simulink library "Energy_converter_Electrical_to_Mechanical"  (R2016a)
settings: Solver=ode1  StartTime=0.0  StopTime=Inf  FixedStep=0.001  RelTol=1e-3
undefined symbols (not defined in the file): API1dcac_efficiency, API2dcac_efficiency, API3dcac_efficiency, aux_power_state, AWR_InvStError, dat, DiscIntNeverNeededParam, EDCU_p_RefTqeMOT, emot_AcCmprFront_inertia, emot_AcCmprFront_nTab_3rdD, emot_AcCmprFront_pwrAC, emot_AcCmprFront_Tau, emot_AcCmprFront_trqTab_2ndD, emot_AcCmprFront_vltTab_1stD, emot_AcCmprRear_inertia, emot_AcCmprRear_nTab_3rdD, emot_AcCmprRear_pwrAC, emot_AcCmprRear_Tau, emot_AcCmprRear_trqTab_2ndD, emot_AcCmprRear_vltTab_1stD, emot_AirCmpr_inertia, emot_AirCmpr_nTab_3rdD, emot_AirCmpr_pwrAC, emot_AirCmpr_Tau, emot_AirCmpr_trqTab_2ndD, emot_AirCmpr_vltTab_1stD, emot_aircomp_power, emot_Cth_rotor, emot_Cth_stator, emot_dtrqEmotNeg, emot_dtrqEmotPtv, emot_inv_pwracTab_1st, emot_inv_pwrDC, emot_inv_pwrLoss, emot_inv_VrmsTab_2nd, emot_j, emot_mot_pwrLoss, emot_nTab_1stD, emot_pwrEtaTab_nRow, emot_pwrEtaTab_pwrTab, emot_pwrEtaTab_trqClm, emot_Rth_rotor_oil, emot_Rth_stator_oil, emot_Rth_stator_rotor, emot_tractiongroup, emot_Trotor_init, emot_trqMaxRow, emot_trqMinRow, emot_Tstator_init, emot_vltTab_3rdD, FirstDrivenAxleNoOfEmot, inv_Cth_cooling_plate, inv_Cth_diode, inv_Cth_IGBT, inv_n_IGBT_per_Switch, inv_Rth_cooling_plate_coolant, inv_Rth_PS_cooling_plate, inv_Tplate_init, inv_Tpowerstack_init, midAxleNoOfEmot ... (+6)
libraries: Electrical_converter x12, Energy_converter_Electrical_to_Mechanical x12, simulink x7
(part 8 of 8)

== system Energy_converter_Electrical_to_Mechanical/e-Motor_chy_proposal/Umrichter mit trq-Regler/Rate Limiter Dynamic/Saturation Dynamic ==
  up : Inport
  u : Inport  Port=2
  lo : Inport  Port=3
  Data Type Duplicate : DataTypeDuplicate  DisableCoverage=on
  Data Type Propagation : S-Function  FunctionName=sfix_dtprop  Parameters=14,PropDataTypeMode,(getdatatypespecs(PropDataType,PropScaling,DblOver,0, 0, PropDataTypeMode, PropScalingMode)),IfRefDouble,IfRefSingle,IsSigned,NumBitsBase,NumBitsMult,NumBitsAdd,(sort(reshape(round(NumBitsAllowFinal), prod(size(NumBitsAllowFinal)),1))),PropScalingMode,ValuesUsedBestPrec,SlopeBase,SlopeMult,SlopeAdd,BiasBase,BiasMult,BiasAdd,DblOver  SFunctionDeploymentMode=off  EnableBusSupport=off  mask(Data Type Propagation){PropDataTypeMode=Inherit via propagation rule, PropDataType=fixdt(1, 16), IfRefDouble=double, IfRefSingle=single, IsSigned=IsSigned1, NumBitsBase=NumBits1, NumBitsMult=1, NumBitsAdd=0, NumBitsAllowFinal=1:128, PropScalingMode=Inherit via propagation rule, PropScaling=2^-10, ValuesUsedBestPrec=[5 -7], SlopeBase=Slope1, SlopeMult=1, SlopeAdd=0, BiasBase=Bias1, BiasMult=1, BiasAdd=0}
      mask prompts: PropDataTypeMode "Simulink:masks:x1PropagatedDataType_MP"; PropDataType "Simulink:masks:x11PropagatedDataTypeegFixdt116Fixdtsingle_MP"; IfRefDouble "Simulink:masks:x11IfAnyReferenceInputIsDoubleOutputIs_MP"; IfRefSingle "Simulink:masks:x12IfAnyReferenceInputIsSingleOutputIs_MP"; IsSigned "Simulink:masks:x13IsSigned_MP"; NumBitsBase "Simulink:masks:x141NumberofBitsBase_MP"; NumBitsMult "Simulink:masks:x142NumberofBitsMultiplicativeAdjustment_MP"; NumBitsAdd "Simulink:masks:x143NumberofBitsAdditiveAdjustment_MP"; NumBitsAllowFinal "Simulink:masks:x144NumberofBitsAllowableFinalValues_MP"; PropScalingMode "Simulink:masks:x2PropagatedScaling_MP"; PropScaling "Simulink:masks:x21PropagatedScalingSlopeEg29OrSlopeBiasEg1253_MP"; ValuesUsedBestPrec "Simulink:masks:x21ValuesUsedToDetermineBestPrecisionScaling_MP"; SlopeBase "Simulink:masks:x211SlopeBase_MP"; SlopeMult "Simulink:masks:x212SlopeMultiplicativeAdjustment_MP"; SlopeAdd "Simulink:masks:x213SlopeAdditiveAdjustment_MP"; BiasBase "Simulink:masks:x221BiasBase_MP"; BiasMult "Simulink:masks:x222BiasMultiplicativeAdjustment_MP"; BiasAdd "Simulink:masks:x223BiasAdditiveAdjustment_MP"
      mask help: Simulink:masks:DataTypePropagation_MD
      mask init:
      | DblOver = 0;
      mask TypeOptions PropDataTypeMode: Simulink:masks:SpecifyViaDialog | Simulink:masks:InheritViaPropagationRule
      mask Callback PropDataTypeMode: fixptdialog(gcbh)
      mask Callback PropDataType: fixptdialog(gcbh)
      mask TypeOptions IfRefDouble: Simulink:masks:double | Simulink:masks:single
      mask TypeOptions IfRefSingle: Simulink:masks:double | Simulink:masks:single
      mask TypeOptions IsSigned: Simulink:masks:IsSigned1 | Simulink:masks:IsSigned2 | Simulink:masks:IsSigned1OrIsSigned2 | Simulink:masks:TRUE | Simulink:masks:FALSE
      mask TypeOptions NumBitsBase: NumBits1 | NumBits2 | max([NumBits1 NumBits2]) | min([NumBits1 NumBits2]) | NumBits1+NumBits2
      mask TypeOptions PropScalingMode: Simulink:masks:SpecifyViaDialog | Simulink:masks:InheritViaPropagationRule | Simulink:masks:ObtainViaBestPrecision
      mask Callback PropScalingMode: fixptdialog(gcbh)
      mask TypeOptions SlopeBase: Slope1 | Slope2 | max([Slope1 Slope2]) | min([Slope1 Slope2]) | Slope1*Slope2 | Slope1/Slope2 | PosRange1 | PosRange2 | max([PosRange1 PosRange2]) | min([PosRange1 PosRange2]) | PosRange1*PosRange2 | PosRange1/PosRange2
      mask TypeOptions BiasBase: Bias1 | Bias2 | max([Bias1 Bias2]) | min([Bias1 Bias2]) | Bias1*Bias2 | Bias1/Bias2 | Bias1+Bias2 | Bias1-Bias2
      mask Display:
      | port_label('Input',1,'Ref1');
      | port_label('Input',2,'Ref2');
      | port_label('Input',3,'Prop');
  LowerRelop1 : RelationalOperator  DisableCoverage=on  Operator=>  OutDataTypeStr=boolean
  Switch : Switch  Criteria=u2 ~= 0  OutDataTypeStr=Inherit: Inherit via back propagation  ZeroCross=off
  Switch2 : Switch  Criteria=u2 ~= 0  OutMin=OutMin  OutMax=OutMax  OutDataTypeStr=Inherit: Inherit via back propagation  ZeroCross=off
  UpperRelop : RelationalOperator  DisableCoverage=on  Operator=<  OutDataTypeStr=boolean
  y : Outport  OutMin=OutMin  OutMax=OutMax
  wires:
  up/1 -> Switch2/1, LowerRelop1/2
  u/1 -> Data Type Propagation/2, Data Type Propagation/1, LowerRelop1/1, Switch/3, UpperRelop/1
  lo/1 -> Switch/1, UpperRelop/2
  Switch/1 -> Data Type Duplicate/2, Switch2/3, Data Type Propagation/3
  Switch2/1 -> Data Type Duplicate/1, y/1
  LowerRelop1/1 -> Switch2/2
  UpperRelop/1 -> Switch/2

== matlab function Energy_converter_Electrical_to_Mechanical/AWR_DriveEmot_Gen2/MotorSelection/Truth Table ==
  data: u1 input; y1 output; u2 input; y2 output; y3 output; y4 output
function [y1, y2, y3, y4] = fcn(u1, u2)

aVarTruthTableCondition_1 = false;
aVarTruthTableCondition_2 = false;
aVarTruthTableCondition_3 = false;
aVarTruthTableCondition_4 = false;
aVarTruthTableCondition_5 = false;
aVarTruthTableCondition_6 = false;
aVarTruthTableCondition_7 = false;
aVarTruthTableCondition_8 = false;
aVarTruthTableCondition_9 = false;


% MidAxle - 0  and Rear Axle - 0 [One Powered Axle]

aVarTruthTableCondition_1 = logical(u1 == 0 && u2 == 0);

% MidAxle - 0  and Rear Axle - 1 [One Powered Axle]

aVarTruthTableCondition_2 = logical(u1 == 0 && u2 == 1);

% MidAxle - 0  and Rear Axle - 2 [One Powered Axle]

aVarTruthTableCondition_3 = logical(u1 == 0 && u2 == 2);

% MidAxle - 1  and Rear Axle - 0 [Two Powered Axle]

aVarTruthTableCondition_4 = logical(u1 == 1 && u2 == 0);

% MidAxle - 1  and Rear Axle - 1 [Two Powered Axle]

aVarTruthTableCondition_5 = logical(u1 == 1 && u2 == 1);

% MidAxle - 1  and Rear Axle - 2 [Two Powered Axle]

aVarTruthTableCondition_6 = logical(u1 == 1 && u2 == 2);

% MidAxle - 2  and Rear Axle - 0 [Two Powered Axle]

aVarTruthTableCondition_7 = logical(u1 == 2 && u2 == 0);

% MidAxle - 2  and Rear Axle - 1 [Two Powered Axle]

aVarTruthTableCondition_8 = logical(u1 == 2 && u2 == 1);

% MidAxle - 2  and Rear Axle - 2 [Two Powered Axle]

aVarTruthTableCondition_9 = logical(u1 == 2 && u2 == 2);

if (aVarTruthTableCondition_1 && ~aVarTruthTableCondition_2 && ~aVarTruthTableCondition_3 && ~aVarTruthTableCondition_4 && ~aVarTruthTableCondition_5 && ~aVarTruthTableCondition_6 && ~aVarTruthTableCondition_7 && ~aVarTruthTableCondition_8 && ~aVarTruthTableCondition_9)
    aFcnTruthTableAction_1();
elseif (~aVarTruthTableCondition_1 && aVarTruthTableCondition_2 && ~aVarTruthTableCondition_3 && ~aVarTruthTableCondition_4 && ~aVarTruthTableCondition_5 && ~aVarTruthTableCondition_6 && ~aVarTruthTableCondition_7 && ~aVarTruthTableCondition_8 && ~aVarTruthTableCondition_9)
    aFcnTruthTableAction_2();
elseif (~aVarTruthTableCondition_1 && ~aVarTruthTableCondition_2 && aVarTruthTableCondition_3 && ~aVarTruthTableCondition_4 && ~aVarTruthTableCondition_5 && ~aVarTruthTableCondition_6 && ~aVarTruthTableCondition_7 && ~aVarTruthTableCondition_8 && ~aVarTruthTableCondition_9)
    aFcnTruthTableAction_3();
elseif (~aVarTruthTableCondition_1 && ~aVarTruthTableCondition_2 && ~aVarTruthTableCondition_3 && aVarTruthTableCondition_4 && ~aVarTruthTableCondition_5 && ~aVarTruthTableCondition_6 && ~aVarTruthTableCondition_7 && ~aVarTruthTableCondition_8 && ~aVarTruthTableCondition_9)
    aFcnTruthTableAction_4();
elseif (~aVarTruthTableCondition_1 && ~aVarTruthTableCondition_2 && ~aVarTruthTableCondition_3 && ~aVarTruthTableCondition_4 && aVarTruthTableCondition_5 && ~aVarTruthTableCondition_6 && ~aVarTruthTableCondition_7 && ~aVarTruthTableCondition_8 && ~aVarTruthTableCondition_9)
    aFcnTruthTableAction_5();
elseif (~aVarTruthTableCondition_1 && ~aVarTruthTableCondition_2 && ~aVarTruthTableCondition_3 && ~aVarTruthTableCondition_4 && ~aVarTruthTableCondition_5 && aVarTruthTableCondition_6 && ~aVarTruthTableCondition_7 && ~aVarTruthTableCondition_8 && ~aVarTruthTableCondition_9)
    aFcnTruthTableAction_6();
elseif (~aVarTruthTableCondition_1 && ~aVarTruthTableCondition_2 && ~aVarTruthTableCondition_3 && ~aVarTruthTableCondition_4 && ~aVarTruthTableCondition_5 && ~aVarTruthTableCondition_6 && aVarTruthTableCondition_7 && ~aVarTruthTableCondition_8 && ~aVarTruthTableCondition_9)
    aFcnTruthTableAction_7();
elseif (~aVarTruthTableCondition_1 && ~aVarTruthTableCondition_2 && ~aVarTruthTableCondition_3 && ~aVarTruthTableCondition_4 && ~aVarTruthTableCondition_5 && ~aVarTruthTableCondition_6 && ~aVarTruthTableCondition_7 && aVarTruthTableCondition_8 && ~aVarTruthTableCondition_9)
    aFcnTruthTableAction_8();
elseif (~aVarTruthTableCondition_1 && ~aVarTruthTableCondition_2 && ~aVarTruthTableCondition_3 && ~aVarTruthTableCondition_4 && ~aVarTruthTableCondition_5 && ~aVarTruthTableCondition_6 && ~aVarTruthTableCondition_7 && ~aVarTruthTableCondition_8 && aVarTruthTableCondition_9)
    aFcnTruthTableAction_9();
else % Default
    aFcnTruthTableAction_10();
end

function aFcnTruthTableAction_1()

% Mid Axle  - NA
% Rear Axle - NA

y1 = 0;
y2 = 0;
y3 = 0;
y4 = 0;

function aFcnTruthTableAction_2()

% Mid Axle  - NA
% Rear Axle - Emot!

y1 = 1;
y2 = 0;
y3 = 0;
y4 = 0;

function aFcnTruthTableAction_3()

% Mid Axle  - NA
% Rear Axle - Emot1 + Emot4

y1 = 1;
y2 = 0;
y3 = 0;
y4 = 1;

function aFcnTruthTableAction_4()

% Mid Axle  - Emot1
% Rear Axle - 0

y1 = 1;
y2 = 0;
y3 = 0;
y4 = 0;

function aFcnTruthTableAction_5()

% Mid Axle  - Emot1
% Rear Axle - Emot3

y1 = 1;
y2 = 0;
y3 = 1;
y4 = 0;

function aFcnTruthTableAction_6()

% Mid Axle  - Emot1
% Rear Axle - Emot3 + Emot4

y1 = 1;
y2 = 0;
y3 = 1;
y4 = 1;

function aFcnTruthTableAction_7()

% Mid Axle  - Emot1 + Emot2
% Rear Axle - 0

y1 = 1;
y2 = 1;
y3 = 0;
y4 = 0;

function aFcnTruthTableAction_8()

% Mid Axle  - Emot1 + Emot2
% Rear Axle - Emot3

y1 = 1;
y2 = 1;
y3 = 1;
y4 = 0;

function aFcnTruthTableAction_9()

% Mid Axle  - Emot1 + Emot2
% Rear Axle - Emot3 + Emot4

y1 = 1;
y2 = 1;
y3 = 1;
y4 = 1;

function aFcnTruthTableAction_10()

% Default

y1 = 0;
y2 = 0;
y3 = 0;
y4 = 0;

== matlab function Energy_converter_Electrical_to_Mechanical/AWR_DriveEmot/MotorSelection/Truth Table ==
  data: u1 input; y1 output; u2 input; y2 output; y3 output; y4 output
function [y1, y2, y3, y4] = fcn(u1, u2)

aVarTruthTableCondition_1 = false;
aVarTruthTableCondition_2 = false;
aVarTruthTableCondition_3 = false;
aVarTruthTableCondition_4 = false;
aVarTruthTableCondition_5 = false;
aVarTruthTableCondition_6 = false;
aVarTruthTableCondition_7 = false;
aVarTruthTableCondition_8 = false;
aVarTruthTableCondition_9 = false;


% 1stDrivenAxle - 0  and 2ndDrivenAxle - 0 [Not Valid]

aVarTruthTableCondition_1 = logical(u1 == 0 && u2 == 0);

% 1stDrivenAxle - 0  and 2ndDrivenAxle - 1 [Not Valid]

aVarTruthTableCondition_2 = logical(u1 == 0 && u2 == 1);

% 1stDrivenAxle - 0  and 2ndDrivenAxle - 2 [Not Valid]

aVarTruthTableCondition_3 = logical(u1 == 0 && u2 == 2);

% 1stDrivenAxle - 1  and 2ndDrivenAxle - 0 [Emot1,-]

aVarTruthTableCondition_4 = logical(u1 == 1 && u2 == 0);

% 1stDrivenAxle - 1  and 2ndDrivenAxle - 1 [Emot1, Emot3]

aVarTruthTableCondition_5 = logical(u1 == 1 && u2 == 1);

% 1stDrivenAxle - 1  and 2ndDrivenAxle - 2 [Emot1, Emot3+Emot4]

aVarTruthTableCondition_6 = logical(u1 == 1 && u2 == 2);

% 1stDrivenAxle - 2  and 2ndDrivenAxle - 0 [Emot1+Emot2,-]

aVarTruthTableCondition_7 = logical(u1 == 2 && u2 == 0);

% 1stDrivenAxle - 2  and 2ndDrivenAxle - 1 [Emot1+Emot2,Emot3]

aVarTruthTableCondition_8 = logical(u1 == 2 && u2 == 1);

% 1stDrivenAxle - 2  and2ndDrivenAxle - 2 [Emot1+Emot2,Emot3+Emot4]

aVarTruthTableCondition_9 = logical(u1 == 2 && u2 == 2);

if (aVarTruthTableCondition_1 && ~aVarTruthTableCondition_2 && ~aVarTruthTableCondition_3 && ~aVarTruthTableCondition_4 && ~aVarTruthTableCondition_5 && ~aVarTruthTableCondition_6 && ~aVarTruthTableCondition_7 && ~aVarTruthTableCondition_8 && ~aVarTruthTableCondition_9)
    aFcnTruthTableAction_1();
elseif (~aVarTruthTableCondition_1 && aVarTruthTableCondition_2 && ~aVarTruthTableCondition_3 && ~aVarTruthTableCondition_4 && ~aVarTruthTableCondition_5 && ~aVarTruthTableCondition_6 && ~aVarTruthTableCondition_7 && ~aVarTruthTableCondition_8 && ~aVarTruthTableCondition_9)
    aFcnTruthTableAction_2();
elseif (~aVarTruthTableCondition_1 && ~aVarTruthTableCondition_2 && aVarTruthTableCondition_3 && ~aVarTruthTableCondition_4 && ~aVarTruthTableCondition_5 && ~aVarTruthTableCondition_6 && ~aVarTruthTableCondition_7 && ~aVarTruthTableCondition_8 && ~aVarTruthTableCondition_9)
    aFcnTruthTableAction_3();
elseif (~aVarTruthTableCondition_1 && ~aVarTruthTableCondition_2 && ~aVarTruthTableCondition_3 && aVarTruthTableCondition_4 && ~aVarTruthTableCondition_5 && ~aVarTruthTableCondition_6 && ~aVarTruthTableCondition_7 && ~aVarTruthTableCondition_8 && ~aVarTruthTableCondition_9)
    aFcnTruthTableAction_4();
elseif (~aVarTruthTableCondition_1 && ~aVarTruthTableCondition_2 && ~aVarTruthTableCondition_3 && ~aVarTruthTableCondition_4 && aVarTruthTableCondition_5 && ~aVarTruthTableCondition_6 && ~aVarTruthTableCondition_7 && ~aVarTruthTableCondition_8 && ~aVarTruthTableCondition_9)
    aFcnTruthTableAction_5();
elseif (~aVarTruthTableCondition_1 && ~aVarTruthTableCondition_2 && ~aVarTruthTableCondition_3 && ~aVarTruthTableCondition_4 && ~aVarTruthTableCondition_5 && aVarTruthTableCondition_6 && ~aVarTruthTableCondition_7 && ~aVarTruthTableCondition_8 && ~aVarTruthTableCondition_9)
    aFcnTruthTableAction_6();
elseif (~aVarTruthTableCondition_1 && ~aVarTruthTableCondition_2 && ~aVarTruthTableCondition_3 && ~aVarTruthTableCondition_4 && ~aVarTruthTableCondition_5 && ~aVarTruthTableCondition_6 && aVarTruthTableCondition_7 && ~aVarTruthTableCondition_8 && ~aVarTruthTableCondition_9)
    aFcnTruthTableAction_7();
elseif (~aVarTruthTableCondition_1 && ~aVarTruthTableCondition_2 && ~aVarTruthTableCondition_3 && ~aVarTruthTableCondition_4 && ~aVarTruthTableCondition_5 && ~aVarTruthTableCondition_6 && ~aVarTruthTableCondition_7 && aVarTruthTableCondition_8 && ~aVarTruthTableCondition_9)
    aFcnTruthTableAction_8();
elseif (~aVarTruthTableCondition_1 && ~aVarTruthTableCondition_2 && ~aVarTruthTableCondition_3 && ~aVarTruthTableCondition_4 && ~aVarTruthTableCondition_5 && ~aVarTruthTableCondition_6 && ~aVarTruthTableCondition_7 && ~aVarTruthTableCondition_8 && aVarTruthTableCondition_9)
    aFcnTruthTableAction_9();
else % Default
    aFcnTruthTableAction_10();
end

function aFcnTruthTableAction_1()

% 1stDrivenAxle - 0 
% 2ndDrivenAxle - 0
% NOT VALID

y1 = 0;
y2 = 0;
y3 = 0;
y4 = 0;

function aFcnTruthTableAction_2()

% 1stDrivenAxle - 0 
% 2ndDrivenAxle - 1
% NOT VALID

y1 = 0;
y2 = 0;
y3 = 0;
y4 = 0;

function aFcnTruthTableAction_3()

% 1stDrivenAxle - 0 
% 2ndDrivenAxle - 2
% NOT VALID

y1 = 0;
y2 = 0;
y3 = 0;
y4 = 0;

function aFcnTruthTableAction_4()

% 1stDrivenAxle - 1 
% 2ndDrivenAxle - 0 [Emot1,-]

y1 = 1;
y2 = 0;
y3 = 0;
y4 = 0;

function aFcnTruthTableAction_5()

% 1stDrivenAxle - 1  
% 2ndDrivenAxle - 1 [Emot1, Emot3]

y1 = 1;
y2 = 0;
y3 = 1;
y4 = 0;

function aFcnTruthTableAction_6()

% 1stDrivenAxle - 1 
% 2ndDrivenAxle - 2 [Emot1, Emot3+Emot4]

y1 = 1;
y2 = 0;
y3 = 1;
y4 = 1;

function aFcnTruthTableAction_7()

% 1stDrivenAxle - 2  
% 2ndDrivenAxle - 0 [Emot1+Emot2,-]

y1 = 1;
y2 = 1;
y3 = 0;
y4 = 0;

function aFcnTruthTableAction_8()

% 1stDrivenAxle - 2  
% 2ndDrivenAxle - 1 [Emot1+Emot2,Emot3]

y1 = 1;
y2 = 1;
y3 = 1;
y4 = 0;

function aFcnTruthTableAction_9()

% 1stDrivenAxle - 2
% 2ndDrivenAxle - 2 [Emot1+Emot2,Emot3+Emot4]

y1 = 1;
y2 = 1;
y3 = 1;
y4 = 1;

function aFcnTruthTableAction_10()

% Default

y1 = 0;
y2 = 0;
y3 = 0;
y4 = 0;
